simulink model "dd_frit_sim"  (R2018b)
settings: Solver=VariableStepAuto  StartTime=0.0  StopTime=endtime  RelTol=1e-3
values from neighbouring files (symbols this model uses):
  db = zeros((endtime-starttime)*epochs + N_0 , nu+ny+1 + 3 + 1)    [Copy_of_dd_pid.m]    (also in Tank_test.m = [[r0(2:endtime+1); zeros(1,1)] r0 y0 [zeros(1,1); y0(1:endti; Tank_test.mat = [100 100 100 100 100 100 100 100 100 100 100 100 ... (5409 e; dd_efrit_pid.m = zeros(N_0 , nu+ny+1 + 3 + 1); dd_frit_pid.m = zeros(N_0 , nu+ny+1 + 3 + 1))
  endtime = 200    [Copy_of_dd_pid.m]    (also in Tank_test.m = 600; Tank_test.mat = 600; dd_efrit_pid.m; dd_frit_pid.m)
  knn = 20    [Copy_of_dd_pid.m]    (also in Tank_test.m = 6; Tank_test.mat = 6; dd_efrit_pid.m = 6; dd_frit_pid.m = 6)
  N_0 = knn + 0    (= 20)    [Copy_of_dd_pid.m]    (also in Tank_test.m = 601; Tank_test.mat = 601; dd_efrit_pid.m = 200; dd_frit_pid.m = 200)
  nu = 2    [Copy_of_dd_pid.m]    (also in Tank_test.m; Tank_test.mat; dd_efrit_pid.m; dd_frit_pid.m)
  ny = 3    [Copy_of_dd_pid.m]    (also in Tank_test.m; Tank_test.mat; dd_efrit_pid.m; dd_frit_pid.m)
  r0 = logsout.getElement('r0').Values.Data    [Tank_test.m]    (also in Tank_test.mat = [100 100 100 100 100 100 100 100 100 100 100 100 ... (601 el; dd_frit_pid_sim.m)
  u0 = zeros(endtime, 1)    [Copy_of_dd_pid.m]    (also in Tank_test.m = logsout.getElement('u0').Values.Data; Tank_test.mat = [10 10 11.9819086502 10.4179804383 11.5257623543 11.25884187; dd_efrit_pid.m; dd_frit_pid.m)
  y0 = zeros(endtime, 1)    [Copy_of_dd_pid.m]    (also in Tank_test.m = logsout.getElement('y0').Values.Data; Tank_test.mat = [-5.63316178038 -4.2765881424 -9.78509931652 -3.53663888787 ; dd_efrit_pid.m; dd_frit_pid.m)
libraries: simulink x1
settings Model: Creator=Tarunbir Singh  LastModifiedBy=Tarunbir Singh

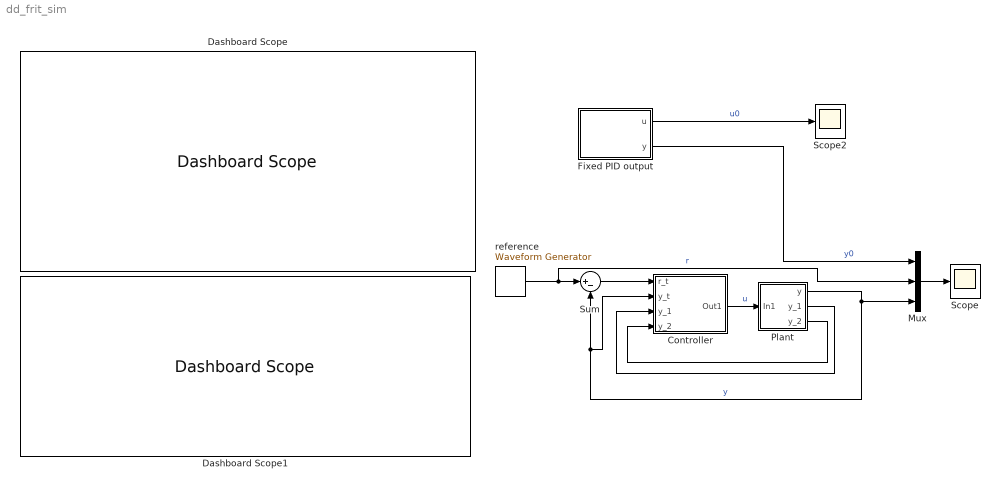
== system dd_frit_sim ==
  "Controller " : Subsystem
  Dashboard Scope : DashboardScope  WebBlockId=36
  Dashboard Scope1 : DashboardScope  WebBlockId=40
  Fixed PID output : MATLAB Function  TreatAsAtomicUnit=on
  Mux : Mux  Inputs=3
  "Plant " : Subsystem
  Scope : Scope
  Scope2 : Scope
  Sum : Sum  Inputs=|+-
  "reference " : simulink/Sources/Waveform Generator  OutMin=[]  OutMax=[]  OutDataTypeStr=double  SelectedSignal=1  Signals=step(0,0,0.5) + step(50,0,0.5) + step(100,0,1) + step(150,0,-0.5)  BlockNames=MultiportSwitch_c8cc2258f1b84cf  SampleTime=1
      settings: SourceProductName=Simulink
  wires:
  "reference "/1 -> Sum/1, Mux/2  "r"
  "Controller "/1(Out1) -> "Plant "/1(In1)  "u"
  Mux/1 -> Scope/1
  "Plant "/1(y) -> Mux/3, "Controller "/2(y_t), Sum/2  "y"
  "Plant "/3(y_2) -> "Controller "/4(y_2)
  "Plant "/2(y_1) -> "Controller "/3(y_1)
  Fixed PID output/2(y) -> Mux/1  "y0"
  Fixed PID output/1(u) -> Scope2/1  "u0"
  Sum/1 -> "Controller "/1(r_t)

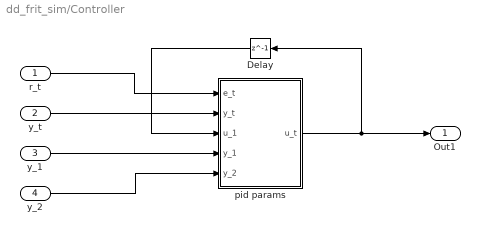
== system dd_frit_sim/Controller  ==
  r_t : Inport
  y_t : Inport  Port=2
  y_1 : Inport  Port=3
  y_2 : Inport  Port=4
  Delay : Delay  DelayLength=1  SampleTime=1
  pid params : MATLAB Function  TreatAsAtomicUnit=on
  Out1 : Outport
  wires:
  r_t/1 -> pid params/1(e_t)
  pid params/1(u_t) -> Out1/1, Delay/1
  y_1/1 -> pid params/4(y_1)
  y_2/1 -> pid params/5(y_2)
  y_t/1 -> pid params/2(y_t)
  Delay/1 -> pid params/3(u_1)

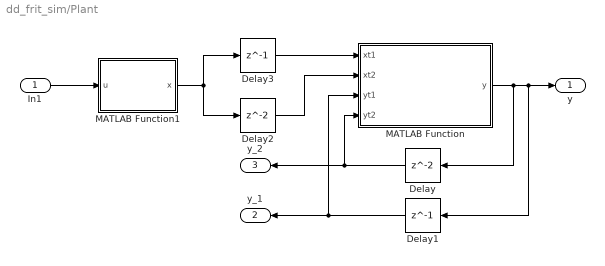
== system dd_frit_sim/Plant  ==
  In1 : Inport
  Delay : Delay  InitialCondition=0  SampleTime=1
  Delay1 : Delay  DelayLength=1  InitialCondition=0  SampleTime=1
  Delay2 : Delay  InitialCondition=0  SampleTime=1
  Delay3 : Delay  DelayLength=1  InitialCondition=0  SampleTime=1
  MATLAB Function : MATLAB Function  TreatAsAtomicUnit=on
  MATLAB Function1 : MATLAB Function  TreatAsAtomicUnit=on
  y : Outport
  y_1 : Outport  Port=2
  y_2 : Outport  Port=3
  wires:
  In1/1 -> MATLAB Function1/1(u)
  MATLAB Function/1(y) -> Delay/1, Delay1/1, y/1
  Delay/1 -> MATLAB Function/4(yt2), y_2/1
  Delay1/1 -> y_1/1, MATLAB Function/3(yt1)
  MATLAB Function1/1(x) -> Delay3/1, Delay2/1
  Delay2/1 -> MATLAB Function/2(xt2)
  Delay3/1 -> MATLAB Function/1(xt1)

== matlab function dd_frit_sim/Plant /MATLAB Function1 ==
  data: u input; x output
function x = fcn(u)

x = 1.5*u - 1.5*u^2 + 0.5*u^3;

== matlab function dd_frit_sim/Plant /MATLAB Function ==
  data: xt1 input; y output; xt2 input; yt1 input; yt2 input
function y = fcn(xt1,xt2,yt1,yt2)

y = 0.6*yt1 - 0.1*yt2 + 1.2*xt1 - 0.1*xt2;

== matlab function dd_frit_sim/Controller /pid params ==
  data: e_t input size=1; y_t input size=1; u_t output; u_1 input size=1; y_1 input size=1; y_2 input size=1; N_0 parameter size=1; r0 parameter size=201; nu parameter size=1; ny parameter size=1; db parameter; knn parameter; endtime parameter
function u_t = fcn(e_t, y_t, u_1, y_1, y_2, N_0, r0, nu, ny, db, knn, endtime)

persistent t 

if isempty(t)
    t = 1;
else
    t = t+1;
end

d_t = zeros(1, N_0);

%% finding nearest neighbours
% information vector / Query

if(t<=endtime)
    query_t = [r0(t+1); r0(t); y_t; y_1; y_2; u_1].';
else
    query_t = [0; r0(t); y_t; y_1; y_2; u_1].';
end
    
    

% k nearest neighbours
for j = 1:N_0
    
    d_t(j) = sum(abs((query_t - db(j,1:nu+ny+1))./(max(db(1:N_0,1:nu+ny+1)) - min(db(1:N_0,1:nu+ny+1)))));
    
end

[~, sorted_index] = sort(d_t);

K_nn = sorted_index(1:knn);

%% Step 3 : Computing PID Parameters

wi_t = exp(-d_t(K_nn))/sum(exp(-d_t(K_nn)));

K = wi_t*db(K_nn, nu+ny+2:nu+ny+4);

u_t = u_1 + K(2)*e_t - K(1)*(y_t - y_1) - K(3)*(y_t - 2*y_1 + y_2);

== matlab function dd_frit_sim/Fixed PID output ==
  data: y0 parameter; u output; y output; u0 parameter
function [u, y] = fcn(y0, u0)

persistent y_0 u_0

if isempty(y_0)
    y_0 = y0;
    u_0 = u0;
else
    y_0 = circshift(y_0, -1, 1);
    u_0 = circshift(u_0, -1, 1);
end
    
y = y_0(1);
u = u_0(1);
